simulink model "VxSpdEsti"  (R2022b)
settings: Solver=VariableStepAuto  StartTime=0.0  StopTime=10.0  RelTol=1e-3
undefined symbols (not defined in the file): Ldwf, Ldwr, thr1, thr2, thr3, TrqRquRate
libraries: simulink x16
settings Model: Creator=YJR  LastModifiedBy=12045

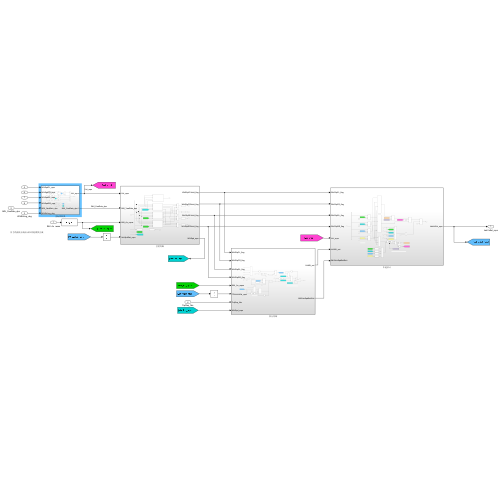
[thumbnail: Simulink's stored preview of the top-level diagram]
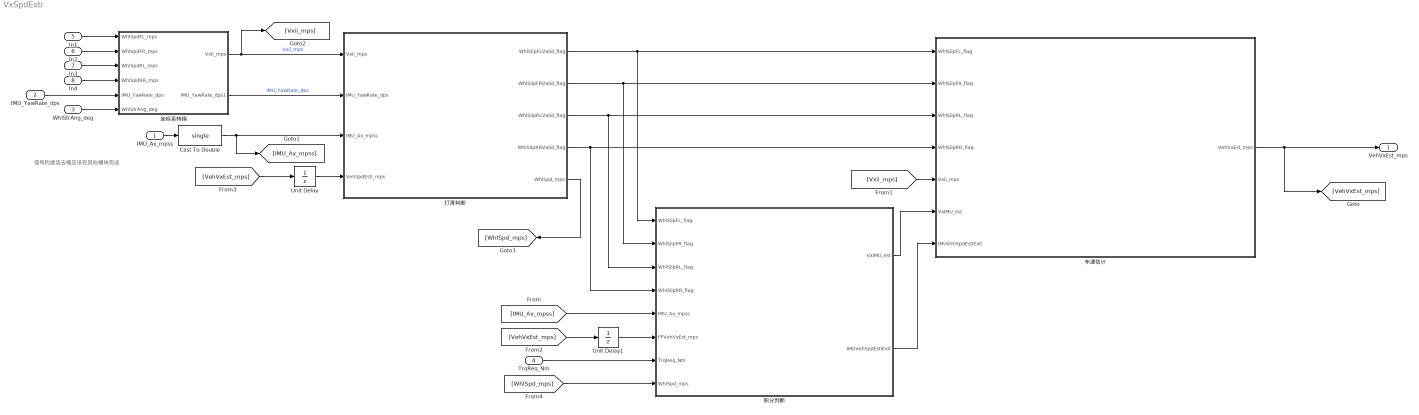
== system VxSpdEsti ==
  note: 信号的滤波去噪应该在其他模块完成
  IMU_Ax_mpss : Inport
  IMU_YawRate_dps : Inport  Port=2
  WhlStrAng_deg : Inport  Port=3
  TrqReq_Nm : Inport  Port=4
  In1 : Inport  Port=5
  In2 : Inport  Port=6
  In3 : Inport  Port=7
  In4 : Inport  Port=8
  Cast To Double : DataTypeConversion  OutDataTypeStr=single  SaturateOnIntegerOverflow=off  RndMeth=Floor
  Unit Delay : UnitDelay  SampleTime=-1  HasFrameUpgradeWarning=on
  Unit Delay1 : UnitDelay  SampleTime=-1  HasFrameUpgradeWarning=on
  坐标系转换 : Subsystem
  打滑判断 : Subsystem
  积分判断 : Subsystem
  车速估计 : Subsystem
  VehVxEst_mps : Outport
  wires:
  坐标系转换/1(Vxii_mps) -> [Vxii_mps], 打滑判断/1(Vxii_mps)  "Vxii_mps"
  坐标系转换/2(IMU_YawRate_dps1) -> 打滑判断/2(IMU_YawRate_dps)  "IMU_YawRate_dps"
  IMU_Ax_mpss/1 -> Cast To Double/1
  [VehVxEst_mps] -> Unit Delay/1
  打滑判断/1(WhlSlipFLValid_flag) -> 车速估计/1(WhlSlipFL_flag), 积分判断/1(WhlSlipFL_flag)
  打滑判断/2(WhlSlipFRValid_flag) -> 车速估计/2(WhlSlipFR_flag), 积分判断/2(WhlSlipFR_flag)
  打滑判断/3(WhlSlipRLValid_flag) -> 车速估计/3(WhlSlipRL_flag), 积分判断/3(WhlSlipRL_flag)
  打滑判断/4(WhlSlipRRValid_flag) -> 车速估计/4(WhlSlipRR_flag), 积分判断/4(WhlSlipRR_flag)
  [IMU_Ax_mpss] -> 积分判断/5(IMU_Ax_mpss)
  积分判断/1(VxIMU_est) -> 车速估计/6(VxIMU_est)
  [Vxii_mps] -> 车速估计/5(Vxii_mps)
  车速估计/1(VehVxEst_mps) -> VehVxEst_mps/1, [VehVxEst_mps]
  [VehVxEst_mps] -> Unit Delay1/1
  Unit Delay/1 -> 打滑判断/4(VehSpdEsti_mps)
  Unit Delay1/1 -> 积分判断/6(FFVehVxEst_mps)
  In1/1 -> 坐标系转换/1(WhlSpdFL_mps)
  In2/1 -> 坐标系转换/2(WhlSpdFR_mps)
  In3/1 -> 坐标系转换/3(WhlSpdRL_mps)
  In4/1 -> 坐标系转换/4(WhlSpdRR_mps)
  IMU_YawRate_dps/1 -> 坐标系转换/5(IMU_YawRate_dps)
  WhlStrAng_deg/1 -> 坐标系转换/6(WhlStrAng_deg)
  TrqReq_Nm/1 -> 积分判断/7(TrqReq_Nm)
  打滑判断/5(WhlSpd_mps) -> [WhlSpd_mps]
  [WhlSpd_mps] -> 积分判断/8(WhlSpd_mps)
  积分判断/2(IMUVehSpdEstiExit) -> 车速估计/7(IMUVehSpdEstiExit)
  Cast To Double/1 -> 打滑判断/3(IMU_Ax_mpss), [IMU_Ax_mpss]

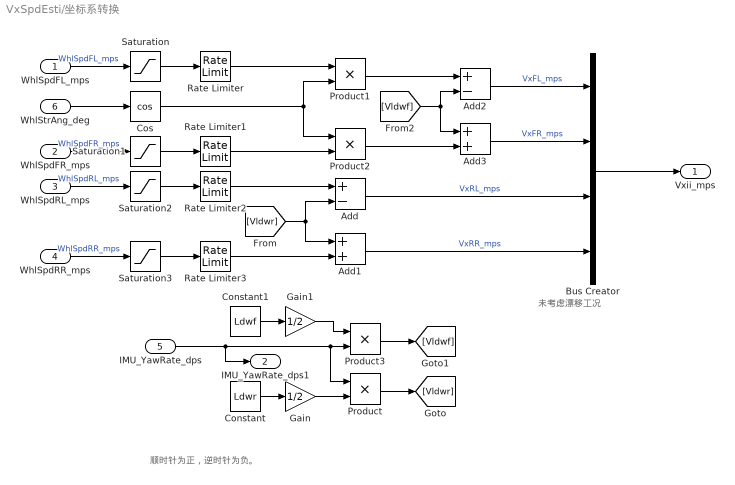
== system VxSpdEsti/坐标系转换 ==
  note: 未考虑漂移工况
  note: 顺时针为正，逆时针为负。
  WhlSpdFL_mps : Inport
  WhlSpdFR_mps : Inport  Port=2
  WhlSpdRL_mps : Inport  Port=3
  WhlSpdRR_mps : Inport  Port=4
  IMU_YawRate_dps : Inport  Port=5
  WhlStrAng_deg : Inport  Port=6
  Add : Sum  Inputs=+-
  Add1 : Sum
  Add2 : Sum  Inputs=+-
  Add3 : Sum
  Bus Creator : BusCreator  Inputs=4
  Constant : Constant  Value=Ldwr
  Constant1 : Constant  Value=Ldwf
  Cos : Trigonometry  Operator=cos
  Gain : Gain  Gain=1/2
  Gain1 : Gain  Gain=1/2
  Product{,1..3} (4 alike) : Product
  Rate Limiter{,1..3} (4 alike) : RateLimiter  SampleTimeMode=inherited
  Saturation{,1..3} (4 alike) : Saturate
  Vxii_mps : Outport
  IMU_YawRate_dps1 : Outport  Port=2
  wires:
  Constant/1 -> Gain/1
  Gain/1 -> Product/2
  IMU_YawRate_dps/1 -> IMU_YawRate_dps1/1, Product/1, Product3/2
  WhlSpdRL_mps/1 -> Saturation2/1  "WhlSpdRL_mps"
  WhlSpdRR_mps/1 -> Saturation3/1  "WhlSpdRR_mps"
  Product/1 -> [Vldwr]
  [Vldwr] -> Add/2, Add1/1
  WhlStrAng_deg/1 -> Cos/1
  WhlSpdFL_mps/1 -> Saturation/1  "WhlSpdFL_mps"
  Cos/1 -> Product1/2, Product2/1
  WhlSpdFR_mps/1 -> Saturation1/1  "WhlSpdFR_mps"
  Constant1/1 -> Gain1/1
  Gain1/1 -> Product3/1
  Product3/1 -> [Vldwf]
  Product1/1 -> Add2/1
  [Vldwf] -> Add2/2, Add3/1
  Product2/1 -> Add3/2
  Add2/1 -> Bus Creator/1  "VxFL_mps"
  Add/1 -> Bus Creator/3  "VxRL_mps"
  Add3/1 -> Bus Creator/2  "VxFR_mps"
  Add1/1 -> Bus Creator/4  "VxRR_mps"
  Bus Creator/1 -> Vxii_mps/1
  Saturation/1 -> Rate Limiter/1
  Saturation1/1 -> Rate Limiter1/1
  Saturation2/1 -> Rate Limiter2/1
  Saturation3/1 -> Rate Limiter3/1
  Rate Limiter/1 -> Product1/1
  Rate Limiter1/1 -> Product2/2
  Rate Limiter2/1 -> Add/1
  Rate Limiter3/1 -> Add1/2

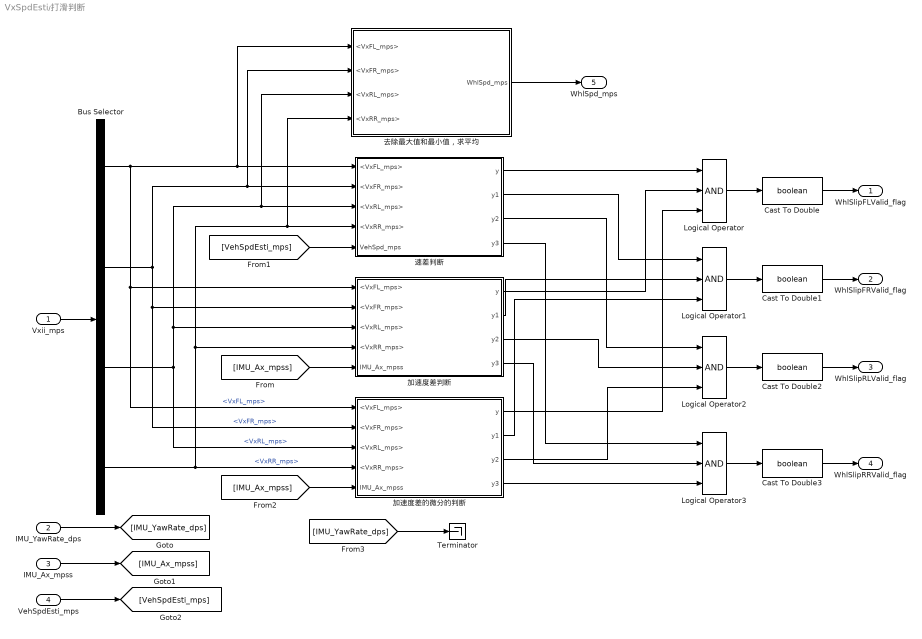
== system VxSpdEsti/打滑判断 ==
  Vxii_mps : Inport
  IMU_YawRate_dps : Inport  Port=2
  IMU_Ax_mpss : Inport  Port=3
  VehSpdEsti_mps : Inport  Port=4
  Bus Selector : BusSelector  OutputSignals=VxFL_mps,VxFR_mps,VxRL_mps,VxRR_mps
  Cast To Double{,1..3} (4 alike) : DataTypeConversion  OutDataTypeStr=boolean  SaturateOnIntegerOverflow=off  RndMeth=Floor
  Logical Operator{,1..3} (4 alike) : Logic  Inputs=3  AllPortsSameDT=off  OutDataTypeStr=boolean
  Terminator : Terminator
  加速度差判断 : Subsystem
  加速度差的微分的判断 : Subsystem
  去除最大值和最小值，求平均 : Subsystem
  速差判断 : Subsystem
  WhlSlipFLValid_flag : Outport
  WhlSlipFRValid_flag : Outport  Port=2
  WhlSlipRLValid_flag : Outport  Port=3
  WhlSlipRRValid_flag : Outport  Port=4
  WhlSpd_mps : Outport  Port=5
  wires:
  速差判断/1(y) -> Logical Operator/1
  加速度差的微分的判断/1(y) -> Logical Operator/3
  加速度差判断/4(y3) -> Logical Operator3/2
  Logical Operator3/1 -> Cast To Double3/1
  Logical Operator2/1 -> Cast To Double2/1
  [IMU_Ax_mpss] -> 加速度差的微分的判断/5(IMU_Ax_mpss)
  加速度差判断/1(y) -> Logical Operator/2
  加速度差的微分的判断/4(y3) -> Logical Operator3/3
  速差判断/2(y1) -> Logical Operator1/1
  [VehSpdEsti_mps] -> 速差判断/5(VehSpd_mps)
  Bus Selector/3 -> 加速度差的微分的判断/3(<VxRL_mps>), 去除最大值和最小值，求平均/3(<VxRL_mps>), 速差判断/3(<VxRL_mps>), 加速度差判断/3(<VxRL_mps>)  "<VxRL_mps>"
  Logical Operator1/1 -> Cast To Double1/1
  加速度差的微分的判断/2(y1) -> Logical Operator1/3
  [IMU_Ax_mpss] -> 加速度差判断/5(IMU_Ax_mpss)
  Bus Selector/4 -> 加速度差判断/4(<VxRR_mps>), 去除最大值和最小值，求平均/4(<VxRR_mps>), 速差判断/4(<VxRR_mps>), 加速度差的微分的判断/4(<VxRR_mps>)  "<VxRR_mps>"
  IMU_YawRate_dps/1 -> [IMU_YawRate_dps]
  Vxii_mps/1 -> Bus Selector/1
  Bus Selector/1 -> 加速度差的微分的判断/1(<VxFL_mps>), 加速度差判断/1(<VxFL_mps>), 去除最大值和最小值，求平均/1(<VxFL_mps>), 速差判断/1(<VxFL_mps>)  "<VxFL_mps>"
  VehSpdEsti_mps/1 -> [VehSpdEsti_mps]
  加速度差的微分的判断/3(y2) -> Logical Operator2/3
  加速度差判断/3(y2) -> Logical Operator2/2
  速差判断/4(y3) -> Logical Operator3/1
  加速度差判断/2(y1) -> Logical Operator1/2
  速差判断/3(y2) -> Logical Operator2/1
  Logical Operator/1 -> Cast To Double/1
  Bus Selector/2 -> 加速度差的微分的判断/2(<VxFR_mps>), 加速度差判断/2(<VxFR_mps>), 去除最大值和最小值，求平均/2(<VxFR_mps>), 速差判断/2(<VxFR_mps>)  "<VxFR_mps>"
  IMU_Ax_mpss/1 -> [IMU_Ax_mpss]
  [IMU_YawRate_dps] -> Terminator/1
  Cast To Double/1 -> WhlSlipFLValid_flag/1
  Cast To Double1/1 -> WhlSlipFRValid_flag/1
  Cast To Double2/1 -> WhlSlipRLValid_flag/1
  Cast To Double3/1 -> WhlSlipRRValid_flag/1
  去除最大值和最小值，求平均/1(WhlSpd_mps) -> WhlSpd_mps/1

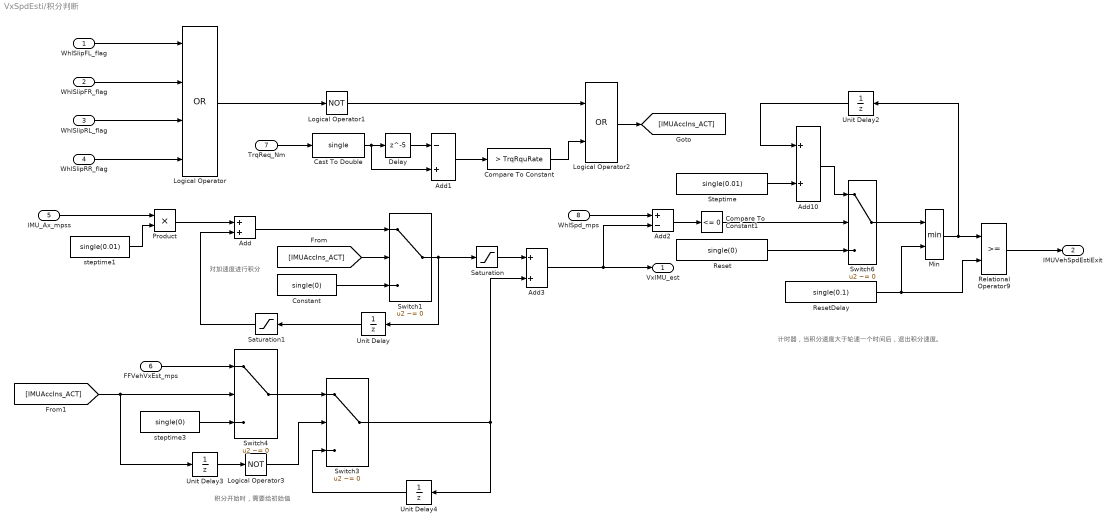
== system VxSpdEsti/积分判断 ==
  note: 对加速度进行积分
  note: 计时器，当积分速度大于轮速一个时间后，退出积分速度。
  note: 积分开始时，需要给初始值
  WhlSlipFL_flag : Inport
  WhlSlipFR_flag : Inport  Port=2
  WhlSlipRL_flag : Inport  Port=3
  WhlSlipRR_flag : Inport  Port=4
  IMU_Ax_mpss : Inport  Port=5
  FFVehVxEst_mps : Inport  Port=6
  TrqReq_Nm : Inport  Port=7
  WhlSpd_mps : Inport  Port=8
  Add : Sum
  Add1 : Sum  Inputs=-+
  Add10 : Sum
  Add2 : Sum  Inputs=+-
  Add3 : Sum
  Cast To Double : DataTypeConversion  OutDataTypeStr=single  SaturateOnIntegerOverflow=off  RndMeth=Floor
  Compare To Constant : simulink/Logic and Bit Operations/Compare To Constant  relop=>  const=TrqRquRate  OutDataTypeStr=boolean
  Compare To Constant1 : simulink/Logic and Bit Operations/Compare To Constant  relop=<=  const=0  OutDataTypeStr=boolean
  Constant : Constant  Value=single(0)
  Delay : Delay  DelayLength=5
  Logical Operator : Logic  Operator=OR  Inputs=4  AllPortsSameDT=off  OutDataTypeStr=boolean
  Logical Operator1 : Logic  Operator=NOT  AllPortsSameDT=off  OutDataTypeStr=boolean
  Logical Operator2 : Logic  Operator=OR  AllPortsSameDT=off  OutDataTypeStr=boolean
  Logical Operator3 : Logic  Operator=NOT  AllPortsSameDT=off  OutDataTypeStr=boolean
  Min : MinMax  Inputs=2
  Product : Product
  Relational Operator9 : RelationalOperator  OutDataTypeStr=boolean  RndMeth=Simplest  InputSameDT=off
  Reset : Constant  Value=single(0)
  ResetDelay : Constant  Value=single(0.1)
  Saturation : Saturate  UpperLimit=50  LowerLimit=-10
  Saturation1 : Saturate  UpperLimit=50  LowerLimit=-10
  Steptime : Constant  Value=single(0.01)
  Switch{1,3..4,6} (4 alike) : Switch  Criteria=u2 ~= 0  SaturateOnIntegerOverflow=off  InputSameDT=off
  Unit Delay : UnitDelay  SampleTime=-1  HasFrameUpgradeWarning=on
  Unit Delay2 : UnitDelay  SampleTime=-1  HasFrameUpgradeWarning=on
  Unit Delay3 : UnitDelay  SampleTime=0.01  HasFrameUpgradeWarning=on
  Unit Delay4 : UnitDelay  SampleTime=-1  HasFrameUpgradeWarning=on
  steptime1 : Constant  Value=single(0.01)
  steptime3 : Constant  Value=single(0)
  VxIMU_est : Outport
  IMUVehSpdEstiExit : Outport  Port=2
  wires:
  WhlSlipFL_flag/1 -> Logical Operator/1
  WhlSlipFR_flag/1 -> Logical Operator/2
  WhlSlipRL_flag/1 -> Logical Operator/3
  WhlSlipRR_flag/1 -> Logical Operator/4
  Logical Operator/1 -> Logical Operator1/1
  Unit Delay/1 -> Saturation1/1
  Add/1 -> Switch1/1
  Switch1/1 -> Saturation/1, Unit Delay/1
  Constant/1 -> Switch1/3
  Logical Operator1/1 -> Logical Operator2/1
  TrqReq_Nm/1 -> Cast To Double/1
  Delay/1 -> Add1/1
  Add1/1 -> Compare To Constant/1
  Compare To Constant/1 -> Logical Operator2/2
  [IMUAccIns_ACT] -> Switch1/2
  Logical Operator2/1 -> [IMUAccIns_ACT]
  Add2/1 -> Compare To Constant1/1
  WhlSpd_mps/1 -> Add2/1
  Saturation1/1 -> Add/2
  Product/1 -> Add/1
  IMU_Ax_mpss/1 -> Product/1
  steptime1/1 -> Product/2
  Saturation/1 -> Add3/1
  Add3/1 -> Add2/2, VxIMU_est/1
  Switch6/1 -> Min/1
  ResetDelay/1 -> Relational Operator9/2, Min/2
  Compare To Constant1/1 -> Switch6/2
  Add10/1 -> Switch6/1
  Steptime/1 -> Add10/2
  Min/1 -> Relational Operator9/1, Unit Delay2/1
  Reset/1 -> Switch6/3
  Unit Delay2/1 -> Add10/1
  FFVehVxEst_mps/1 -> Switch4/1
  Unit Delay3/1 -> Logical Operator3/1
  steptime3/1 -> Switch4/3
  Logical Operator3/1 -> Switch3/2
  Switch3/1 -> Add3/2, Unit Delay4/1
  Switch4/1 -> Switch3/1
  Cast To Double/1 -> Delay/1, Add1/2
  [IMUAccIns_ACT] -> Unit Delay3/1, Switch4/2
  Unit Delay4/1 -> Switch3/3
  Relational Operator9/1 -> IMUVehSpdEstiExit/1

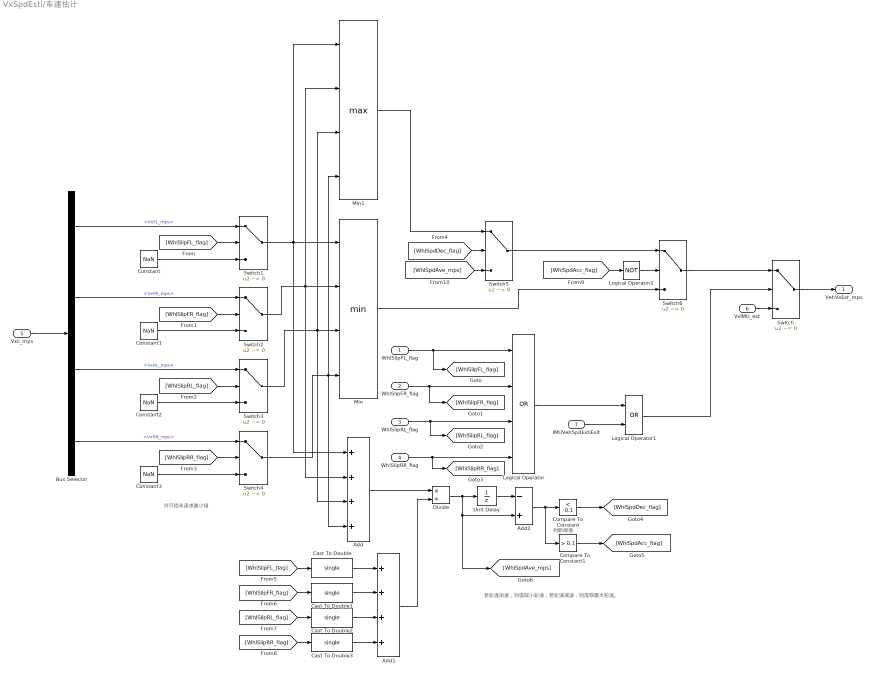
== system VxSpdEsti/车速估计 ==
  note: 若轮速加速，则选取小轮速；若轮速减速，则选取最大轮速。
  note: 判断阈值
  note: 对可信车速求最小值
  WhlSlipFL_flag : Inport
  WhlSlipFR_flag : Inport  Port=2
  WhlSlipRL_flag : Inport  Port=3
  WhlSlipRR_flag : Inport  Port=4
  Vxii_mps : Inport  Port=5
  VxIMU_est : Inport  Port=6
  IMUVehSpdEstiExit : Inport  Port=7
  Add : Sum  Inputs=++++
  Add1 : Sum  Inputs=++++
  Add2 : Sum  Inputs=-+
  Bus Selector : BusSelector  OutputSignals=VxFL_mps,VxFR_mps,VxRL_mps,VxRR_mps
  Cast To Double{,1..3} (4 alike) : DataTypeConversion  OutDataTypeStr=single  SaturateOnIntegerOverflow=off  RndMeth=Floor
  Compare To Constant : simulink/Logic and Bit Operations/Compare To Constant  relop=<  const=-0.1  OutDataTypeStr=boolean
  Compare To Constant1 : simulink/Logic and Bit Operations/Compare To Constant  relop=>  const=0.1  OutDataTypeStr=boolean
  Constant{,1..3} (4 alike) : Constant  Value=NaN
  Divide : Product  Inputs=*/
  Logical Operator : Logic  Operator=OR  Inputs=4  AllPortsSameDT=off  OutDataTypeStr=boolean
  Logical Operator1 : Logic  Operator=OR  AllPortsSameDT=off  OutDataTypeStr=boolean
  Logical Operator2 : Logic  Operator=NOT  AllPortsSameDT=off  OutDataTypeStr=boolean
  Min : MinMax  Inputs=4
  Min1 : MinMax  Function=max  Inputs=4
  Switch{,1..6} (7 alike) : Switch  Criteria=u2 ~= 0  SaturateOnIntegerOverflow=off  InputSameDT=off
  Unit Delay : UnitDelay  SampleTime=-1  HasFrameUpgradeWarning=on
  VehVxEst_mps : Outport
  wires:
  WhlSlipFL_flag/1 -> [WhlSlipFL_flag], Logical Operator/1
  WhlSlipFR_flag/1 -> [WhlSlipFR_flag], Logical Operator/2
  WhlSlipRL_flag/1 -> [WhlSlipRL_flag], Logical Operator/3
  WhlSlipRR_flag/1 -> [WhlSlipRR_flag], Logical Operator/4
  Vxii_mps/1 -> Bus Selector/1
  Bus Selector/1 -> Switch1/1  "<VxFL_mps>"
  Bus Selector/2 -> Switch2/1  "<VxFR_mps>"
  Bus Selector/3 -> Switch3/1  "<VxRL_mps>"
  Bus Selector/4 -> Switch4/1  "<VxRR_mps>"
  VxIMU_est/1 -> Switch/3
  [WhlSlipFL_flag] -> Switch1/2
  Constant/1 -> Switch1/3
  Constant1/1 -> Switch2/3
  [WhlSlipFR_flag] -> Switch2/2
  [WhlSlipRL_flag] -> Switch3/2
  Constant2/1 -> Switch3/3
  Constant3/1 -> Switch4/3
  [WhlSlipRR_flag] -> Switch4/2
  Switch1/1 -> Min/1, Add/1, Min1/1
  Switch2/1 -> Add/2, Min/2, Min1/2
  Switch3/1 -> Min/3, Add/3, Min1/3
  Switch4/1 -> Add/4, Min1/4, Min/4
  Switch/1 -> VehVxEst_mps/1
  Logical Operator/1 -> Logical Operator1/1
  Logical Operator1/1 -> Switch/2
  IMUVehSpdEstiExit/1 -> Logical Operator1/2
  Min1/1 -> Switch5/1
  [WhlSpdDec_flag] -> Switch5/2
  Add/1 -> Divide/1
  [WhlSlipFL_flag] -> Cast To Double/1
  [WhlSlipFR_flag] -> Cast To Double1/1
  [WhlSlipRL_flag] -> Cast To Double2/1
  [WhlSlipRR_flag] -> Cast To Double3/1
  Add1/1 -> Divide/2
  Divide/1 -> Add2/2, [WhlSpdAve_mps], Unit Delay/1
  Unit Delay/1 -> Add2/1
  Add2/1 -> Compare To Constant1/1, Compare To Constant/1
  Compare To Constant/1 -> [WhlSpdDec_flag]
  Switch6/1 -> Switch/1
  Compare To Constant1/1 -> [WhlSpdAcc_flag]
  [WhlSpdAcc_flag] -> Logical Operator2/1
  Switch5/1 -> Switch6/1
  Min/1 -> Switch6/3
  Logical Operator2/1 -> Switch6/2
  [WhlSpdAve_mps] -> Switch5/3
  Cast To Double/1 -> Add1/1
  Cast To Double1/1 -> Add1/2
  Cast To Double2/1 -> Add1/3
  Cast To Double3/1 -> Add1/4

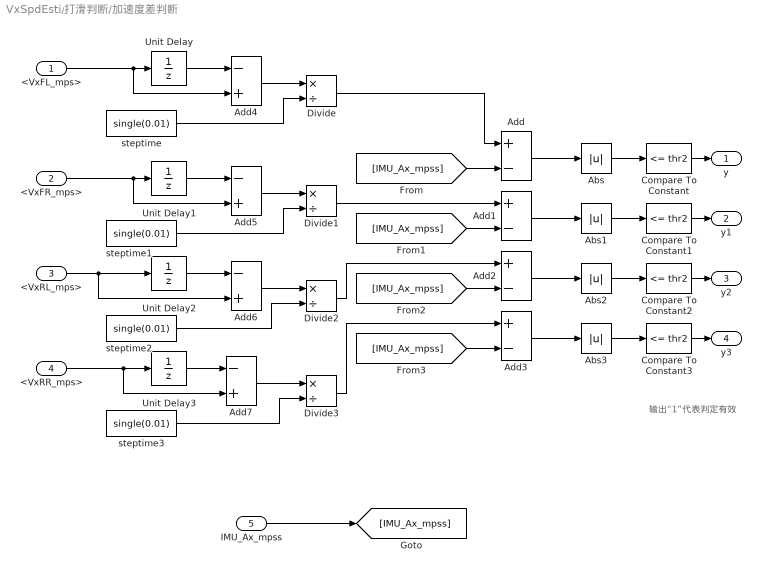
== system VxSpdEsti/打滑判断/加速度差判断 ==
  note: 输出“1”代表判定有效
  <VxFL_mps> : Inport
  <VxFR_mps> : Inport  Port=2
  <VxRL_mps> : Inport  Port=3
  <VxRR_mps> : Inport  Port=4
  IMU_Ax_mpss : Inport  Port=5
  Abs{,1..3} (4 alike) : Abs  SaturateOnIntegerOverflow=off
  Add{,1..3} (4 alike) : Sum  Inputs=+-
  Add{4..7} (4 alike) : Sum  Inputs=-+
  Compare To Constant{,1..3} (4 alike) : simulink/Logic and Bit Operations/Compare To Constant  relop=<=  const=thr2  OutDataTypeStr=boolean
  Divide{,1..3} (4 alike) : Product  Inputs=*/
  Unit Delay{,1..3} (4 alike) : UnitDelay  SampleTime=-1  HasFrameUpgradeWarning=on
  steptime{,1..3} (4 alike) : Constant  Value=single(0.01)
  y : Outport
  y1 : Outport  Port=2
  y2 : Outport  Port=3
  y3 : Outport  Port=4
  wires:
  Compare To Constant/1 -> y/1
  Compare To Constant2/1 -> y2/1
  Abs2/1 -> Compare To Constant2/1
  Add1/1 -> Abs1/1
  Abs/1 -> Compare To Constant/1
  [IMU_Ax_mpss] -> Add3/2
  [IMU_Ax_mpss] -> Add2/2
  [IMU_Ax_mpss] -> Add/2
  Abs3/1 -> Compare To Constant3/1
  Compare To Constant3/1 -> y3/1
  Compare To Constant1/1 -> y1/1
  [IMU_Ax_mpss] -> Add1/2
  Add/1 -> Abs/1
  Add3/1 -> Abs3/1
  Abs1/1 -> Compare To Constant1/1
  Add2/1 -> Abs2/1
  <VxFL_mps>/1 -> Add4/2, Unit Delay/1
  Unit Delay/1 -> Add4/1
  Add4/1 -> Divide/1
  steptime/1 -> Divide/2
  Divide/1 -> Add/1
  IMU_Ax_mpss/1 -> [IMU_Ax_mpss]
  steptime1/1 -> Divide1/2
  Add5/1 -> Divide1/1
  Unit Delay1/1 -> Add5/1
  <VxFR_mps>/1 -> Unit Delay1/1, Add5/2
  Divide1/1 -> Add1/1
  steptime2/1 -> Divide2/2
  Add6/1 -> Divide2/1
  Unit Delay2/1 -> Add6/1
  <VxRL_mps>/1 -> Unit Delay2/1, Add6/2
  Divide2/1 -> Add2/1
  steptime3/1 -> Divide3/2
  Add7/1 -> Divide3/1
  Unit Delay3/1 -> Add7/1
  <VxRR_mps>/1 -> Unit Delay3/1, Add7/2
  Divide3/1 -> Add3/1

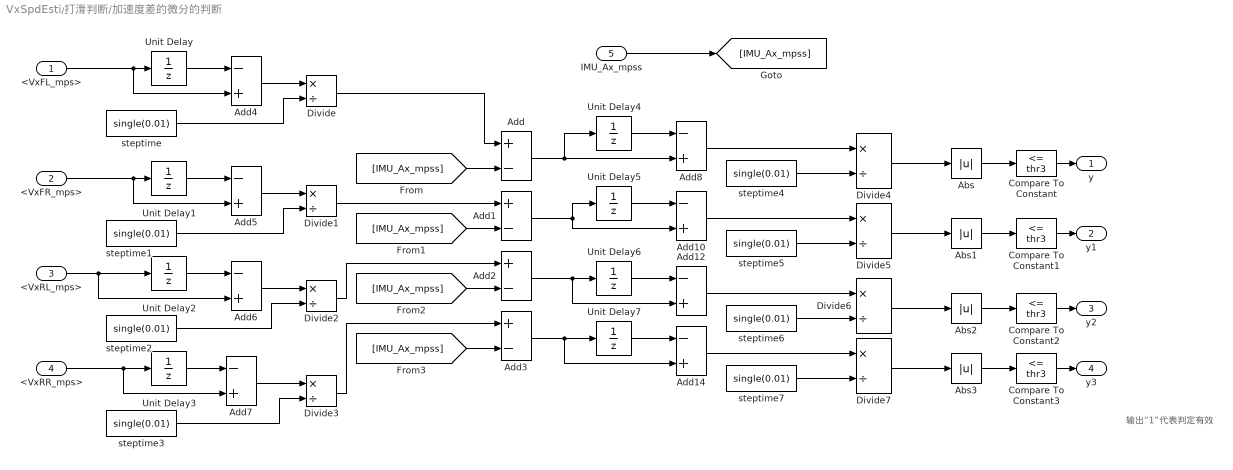
== system VxSpdEsti/打滑判断/加速度差的微分的判断 ==
  note: 输出“1”代表判定有效
  <VxFL_mps> : Inport
  <VxFR_mps> : Inport  Port=2
  <VxRL_mps> : Inport  Port=3
  <VxRR_mps> : Inport  Port=4
  IMU_Ax_mpss : Inport  Port=5
  Abs{,1..3} (4 alike) : Abs  SaturateOnIntegerOverflow=off
  Add{,1..3} (4 alike) : Sum  Inputs=+-
  Add{4..8,10,12,14} (8 alike) : Sum  Inputs=-+
  Compare To Constant{,1..3} (4 alike) : simulink/Logic and Bit Operations/Compare To Constant  relop=<=  const=thr3  OutDataTypeStr=boolean
  Divide{,1..7} (8 alike) : Product  Inputs=*/
  Unit Delay{,1..7} (8 alike) : UnitDelay  SampleTime=-1  HasFrameUpgradeWarning=on
  steptime{,1..7} (8 alike) : Constant  Value=single(0.01)
  y : Outport
  y1 : Outport  Port=2
  y2 : Outport  Port=3
  y3 : Outport  Port=4
  wires:
  Divide3/1 -> Add3/1
  <VxRR_mps>/1 -> Add7/2, Unit Delay3/1
  Unit Delay3/1 -> Add7/1
  Add7/1 -> Divide3/1
  steptime3/1 -> Divide3/2
  Divide2/1 -> Add2/1
  <VxRL_mps>/1 -> Add6/2, Unit Delay2/1
  Unit Delay2/1 -> Add6/1
  Add6/1 -> Divide2/1
  steptime2/1 -> Divide2/2
  Divide1/1 -> Add1/1
  <VxFR_mps>/1 -> Add5/2, Unit Delay1/1
  Unit Delay1/1 -> Add5/1
  Add5/1 -> Divide1/1
  steptime1/1 -> Divide1/2
  IMU_Ax_mpss/1 -> [IMU_Ax_mpss]
  Divide/1 -> Add/1
  steptime/1 -> Divide/2
  Add4/1 -> Divide/1
  Unit Delay/1 -> Add4/1
  <VxFL_mps>/1 -> Unit Delay/1, Add4/2
  Abs1/1 -> Compare To Constant1/1
  [IMU_Ax_mpss] -> Add1/2
  Compare To Constant1/1 -> y1/1
  Compare To Constant3/1 -> y3/1
  Abs3/1 -> Compare To Constant3/1
  [IMU_Ax_mpss] -> Add/2
  [IMU_Ax_mpss] -> Add2/2
  [IMU_Ax_mpss] -> Add3/2
  Abs/1 -> Compare To Constant/1
  Abs2/1 -> Compare To Constant2/1
  Compare To Constant2/1 -> y2/1
  Compare To Constant/1 -> y/1
  Add/1 -> Add8/2, Unit Delay4/1
  Unit Delay4/1 -> Add8/1
  Add8/1 -> Divide4/1
  steptime4/1 -> Divide4/2
  Divide4/1 -> Abs/1
  steptime5/1 -> Divide5/2
  Add10/1 -> Divide5/1
  Unit Delay5/1 -> Add10/1
  Add1/1 -> Unit Delay5/1, Add10/2
  Divide5/1 -> Abs1/1
  Divide6/1 -> Abs2/1
  Add2/1 -> Add12/2, Unit Delay6/1
  Add12/1 -> Divide6/1
  steptime6/1 -> Divide6/2
  Unit Delay6/1 -> Add12/1
  steptime7/1 -> Divide7/2
  Add14/1 -> Divide7/1
  Add3/1 -> Add14/2, Unit Delay7/1
  Unit Delay7/1 -> Add14/1
  Divide7/1 -> Abs3/1

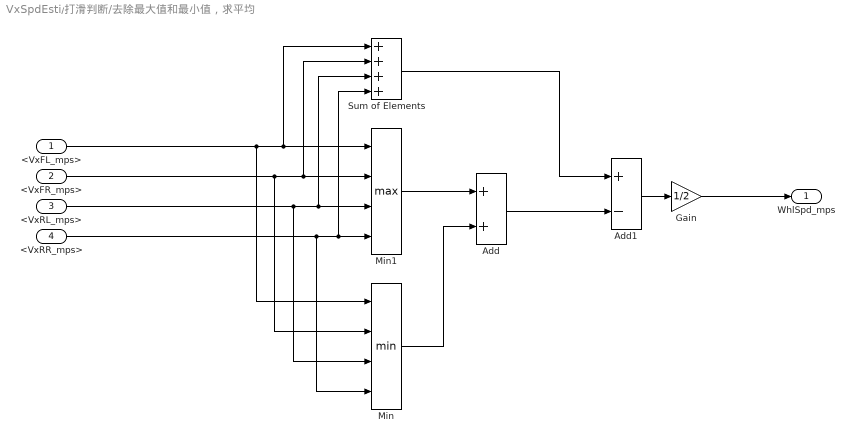
== system VxSpdEsti/打滑判断/去除最大值和最小值，求平均 ==
  <VxFL_mps> : Inport
  <VxFR_mps> : Inport  Port=2
  <VxRL_mps> : Inport  Port=3
  <VxRR_mps> : Inport  Port=4
  Add : Sum
  Add1 : Sum  Inputs=+-
  Gain : Gain  Gain=1/2
  Min : MinMax  Inputs=4
  Min1 : MinMax  Function=max  Inputs=4
  Sum of Elements : Sum  Inputs=++++
  WhlSpd_mps : Outport
  wires:
  Gain/1 -> WhlSpd_mps/1
  Add1/1 -> Gain/1
  <VxRL_mps>/1 -> Min/3, Sum of Elements/3, Min1/3
  <VxFL_mps>/1 -> Min/1, Sum of Elements/1, Min1/1
  Min/1 -> Add/2
  <VxRR_mps>/1 -> Min/4, Sum of Elements/4, Min1/4
  Min1/1 -> Add/1
  Add/1 -> Add1/2
  Sum of Elements/1 -> Add1/1
  <VxFR_mps>/1 -> Min/2, Sum of Elements/2, Min1/2

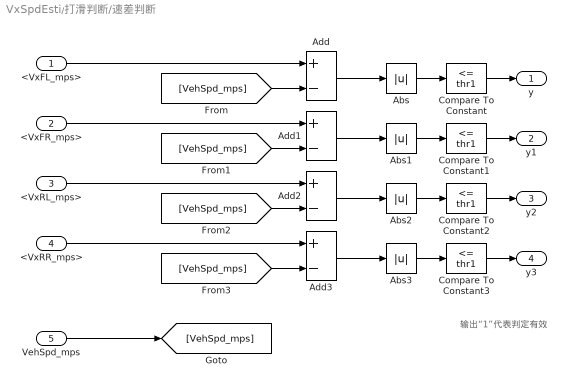
== system VxSpdEsti/打滑判断/速差判断 ==
  note: 输出“1”代表判定有效
  <VxFL_mps> : Inport
  <VxFR_mps> : Inport  Port=2
  <VxRL_mps> : Inport  Port=3
  <VxRR_mps> : Inport  Port=4
  VehSpd_mps : Inport  Port=5
  Abs{,1..3} (4 alike) : Abs  SaturateOnIntegerOverflow=off
  Add{,1..3} (4 alike) : Sum  Inputs=+-
  Compare To Constant{,1..3} (4 alike) : simulink/Logic and Bit Operations/Compare To Constant  relop=<=  const=thr1  OutDataTypeStr=boolean
  y : Outport
  y1 : Outport  Port=2
  y2 : Outport  Port=3
  y3 : Outport  Port=4
  wires:
  Add2/1 -> Abs2/1
  Abs1/1 -> Compare To Constant1/1
  <VxRR_mps>/1 -> Add3/1
  Add3/1 -> Abs3/1
  Add/1 -> Abs/1
  [VehSpd_mps] -> Add1/2
  <VxRL_mps>/1 -> Add2/1
  <VxFR_mps>/1 -> Add1/1
  Compare To Constant1/1 -> y1/1
  Compare To Constant3/1 -> y3/1
  Abs3/1 -> Compare To Constant3/1
  [VehSpd_mps] -> Add/2
  [VehSpd_mps] -> Add2/2
  [VehSpd_mps] -> Add3/2
  Abs/1 -> Compare To Constant/1
  Add1/1 -> Abs1/1
  Abs2/1 -> Compare To Constant2/1
  <VxFL_mps>/1 -> Add/1
  Compare To Constant2/1 -> y2/1
  Compare To Constant/1 -> y/1
  VehSpd_mps/1 -> [VehSpd_mps]
